simulink library "environment_cl"  (R2018b)
settings: Solver=VariableStepAuto  StartTime=0.0  StopTime=10.0  RelTol=1e-3
undefined symbols (not defined in the file or in its folder): initializeBussesFromBlock
libraries: $bdroot x2, flowcalculation_cl x2
settings Model: Creator=mcobb  LastModifiedBy=mcobb

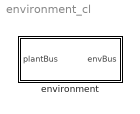
== system environment_cl ==
  environment : Subsystem  LoadFcn=initializeBussesFromBlock(gcb)  InitFcn=initializeBussesFromBlock(gcb)  StartFcn=initializeBussesFromBlock(gcb)
      settings: MinAlgLoopOccurrences=on

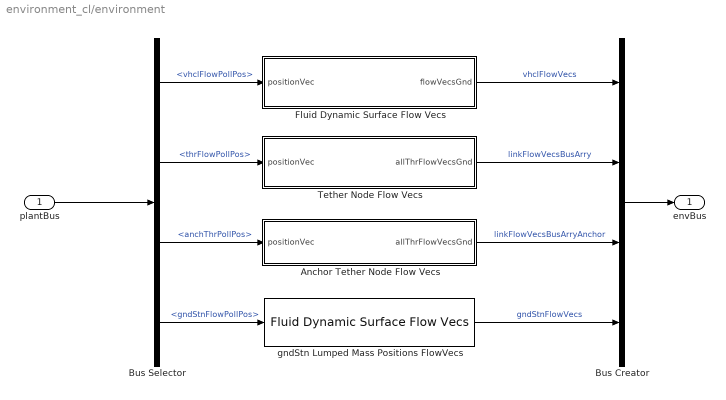
== system environment_cl/environment ==
  plantBus : Inport  OutDataTypeStr=Bus: plantBus
  Anchor Tether Node Flow Vecs : Subsystem
  Bus Creator : BusCreator  Inputs=4  OutDataTypeStr=Bus: envBus  NonVirtualBus=on
  Bus Selector : BusSelector  OutputSignals=vhclFlowPollPos,thrFlowPollPos,anchThrPollPos,gndStnFlowPollPos
  Fluid Dynamic Surface Flow Vecs : Subsystem
      settings: MinAlgLoopOccurrences=on
  Tether Node Flow Vecs : Subsystem
      settings: MinAlgLoopOccurrences=on
  gndStn Lumped Mass Positions FlowVecs : $bdroot/environment/Fluid Dynamic Surface Flow Vecs  SystemSampleTime=-1
  envBus : Outport  OutDataTypeStr=Bus: envBus
  wires:
  Bus Selector/1 -> Fluid Dynamic Surface Flow Vecs/1(positionVec)  "<vhclFlowPollPos>"
  Fluid Dynamic Surface Flow Vecs/1(flowVecsGnd) -> Bus Creator/1  "vhclFlowVecs"
  Tether Node Flow Vecs/1(allThrFlowVecsGnd) -> Bus Creator/2  "linkFlowVecsBusArry"
  Bus Creator/1 -> envBus/1
  Bus Selector/3 -> Anchor Tether Node Flow Vecs/1(positionVec)  "<anchThrPollPos>"
  Anchor Tether Node Flow Vecs/1(allThrFlowVecsGnd) -> Bus Creator/3  "linkFlowVecsBusArryAnchor"
  Bus Selector/2 -> Tether Node Flow Vecs/1(positionVec)  "<thrFlowPollPos>"
  plantBus/1 -> Bus Selector/1
  gndStn Lumped Mass Positions FlowVecs/1 -> Bus Creator/4  "gndStnFlowVecs"
  Bus Selector/4 -> gndStn Lumped Mass Positions FlowVecs/1  "<gndStnFlowPollPos>"

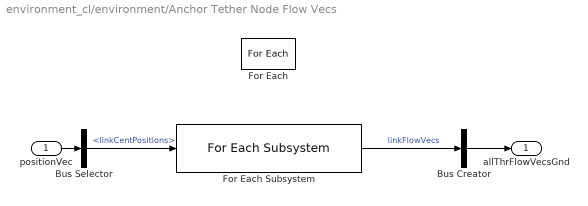
== system environment_cl/environment/Anchor Tether Node Flow Vecs ==
  positionVec : Inport  OutDataTypeStr=Bus: thrPollPosBus  Partition=on  PartitionDimension=1  PartitionWidth=1  PartitionOffset=0
  Bus Creator : BusCreator  Inputs=1  OutDataTypeStr=Bus: linkFlowVecsAnchorBus  NonVirtualBus=on
  Bus Selector : BusSelector  OutputSignals=linkCentPositions
  For Each : ForEach  DisableCoverage=on  IndexMode=One-based
  For Each Subsystem : $bdroot/environment/Tether Node Flow Vecs/For Each Subsystem  SystemSampleTime=-1
  allThrFlowVecsGnd : Outport  OutDataTypeStr=Bus: linkFlowVecsAnchorBus  ConcatenationDimension=1
  wires:
  Bus Selector/1 -> For Each Subsystem/1  "<linkCentPositions>"
  For Each Subsystem/1 -> Bus Creator/1  "linkFlowVecs"
  Bus Creator/1 -> allThrFlowVecsGnd/1
  positionVec/1 -> Bus Selector/1

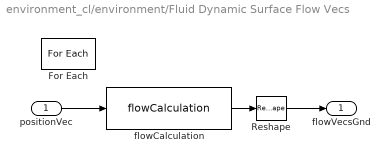
== system environment_cl/environment/Fluid Dynamic Surface Flow Vecs ==
  positionVec : Inport  Partition=on  PartitionDimension=2  PartitionWidth=1  PartitionOffset=0
  For Each : ForEach  DisableCoverage=on  IndexMode=One-based
  Reshape : Reshape  OutputDimensionality=Column vector (2-D)
  flowCalculation : flowcalculation_cl/flowCalculation  SystemSampleTime=-1
  flowVecsGnd : Outport  ConcatenationDimension=2
  wires:
  positionVec/1 -> flowCalculation/1
  flowCalculation/1 -> Reshape/1
  Reshape/1 -> flowVecsGnd/1

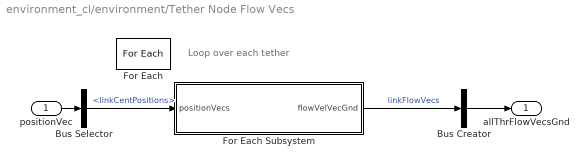
== system environment_cl/environment/Tether Node Flow Vecs ==
  note: Loop over each tether
  positionVec : Inport  Partition=on  PartitionDimension=1  PartitionWidth=1  PartitionOffset=0
  Bus Creator : BusCreator  Inputs=1  OutDataTypeStr=Bus: linkFlowVecsBus  NonVirtualBus=on
  Bus Selector : BusSelector  OutputSignals=linkCentPositions
  For Each : ForEach  DisableCoverage=on  IndexMode=One-based
  For Each Subsystem : Subsystem
      settings: MinAlgLoopOccurrences=on
  allThrFlowVecsGnd : Outport  OutDataTypeStr=Bus: linkFlowVecsBus  ConcatenationDimension=1
  wires:
  positionVec/1 -> Bus Selector/1
  For Each Subsystem/1(flowVelVecGnd) -> Bus Creator/1  "linkFlowVecs"
  Bus Creator/1 -> allThrFlowVecsGnd/1
  Bus Selector/1 -> For Each Subsystem/1(positionVecs)  "<linkCentPositions>"

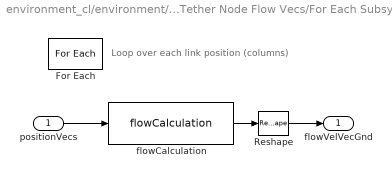
== system environment_cl/environment/Tether Node Flow Vecs/For Each Subsystem ==
  note: Loop over each link position (columns)
  positionVecs : Inport  Partition=on  PartitionDimension=2  PartitionWidth=1  PartitionOffset=0
  For Each : ForEach  DisableCoverage=on  IndexMode=One-based
  Reshape : Reshape  OutputDimensionality=Column vector (2-D)
  flowCalculation : flowcalculation_cl/flowCalculation  SystemSampleTime=-1
  flowVelVecGnd : Outport  ConcatenationDimension=2
  wires:
  flowCalculation/1 -> Reshape/1
  Reshape/1 -> flowVelVecGnd/1
  positionVecs/1 -> flowCalculation/1
